simulink model "matlabFunctionTest1"  (R2023a)
settings: Solver=VariableStepAuto  StartTime=0.0  StopTime=10.0  FixedStep=1  RelTol=1e-3
settings Model: Creator=涂钱龙  LastModifiedBy=涂钱龙

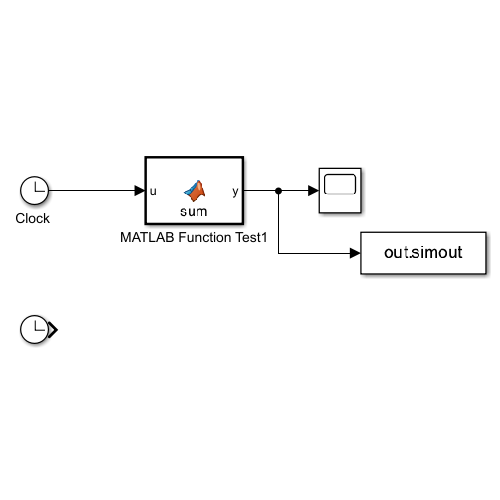
[thumbnail: Simulink's stored preview of the top-level diagram]
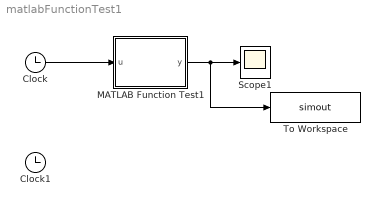
== system matlabFunctionTest1 ==
  "Clock " : Clock
  Clock1 : Clock
  MATLAB Function Test1 : MATLAB Function  TreatAsAtomicUnit=on
  Scope1 : Scope
  To Workspace : ToWorkspace  VariableName=simout  SaveFormat=Timeseries  SampleTime=-1
  wires:
  MATLAB Function Test1/1(y) -> To Workspace/1, Scope1/1
  "Clock "/1 -> MATLAB Function Test1/1(u)

== matlab function matlabFunctionTest1/MATLAB Function Test1 ==
  data: y output; u input
function y = sum(u)
%% 
% u是输入，y是输出
% 要实现对输入的累加
persistent sum_total; % 函数内部声明 持久变量 
% 首先判断 persistent 声明的变量是否为空
if isempty(sum_total)
    sum_total = 0;
end
sum_total = u + sum_total;
y = sum_total;
%%
